simulink model "LOG_DATI_GPS_BMP_07_119_term"  (R2020b)
settings: Solver=ode4  StartTime=0.0  StopTime=Inf  FixedStep=0.02  RelTol=1e-3  EnableMultiTasking=on
PostLoadFcn:
  | , if any(exist('dsrtsu_mdlpostloadfcn', 'file') == [2, 3, 6]), try dsrtsu_mdlpostloadfcn('Execute', bdroot); catch fprintf('Error in PostLoadFcn (dsrtsu_mdlpostloadfcn) for model "%s":\n %s\n', bdroot, lasterr); end, end,
InitFcn:
  | , if any(exist('rtifpga_mdlclblib', 'file') ~= 0), rtifpga_mdlclblib('Init', bdroot); end,
values from neighbouring files (symbols this model uses):
  t_AP = 0.02    [AVVIO_AENEA_DATA.m]    (also in workspace_SFT.mat)
libraries: arduinolib x21, simulink_extras x6, svdutilitieslib x4, simulink x2
(part 3 of 3)

== matlab function LOG_DATI_GPS_BMP_07_119_term/AIR RX/MATLAB Function4 ==
  data: byte_pack input; status output; messaggio output; messaggio_2 output; byte_available input
function [status,messaggio,messaggio_2]  = Creazione_mavlink_message_2(byte_pack,byte_available)


persistent Interr_parz  message counter len_found mess_len

if isempty(Interr_parz)
    Interr_parz = false ;
end
if isempty(message)
     message = uint8(zeros(1,100 )) ;
end
if isempty (counter) 
    counter = uint8(0) ;    % variabile che conta quanti byte mancano per completare il messaggio
end 

if isempty(len_found) 
     len_found = false ;
end 

if isempty(mess_len) 
     mess_len = 0 ;
end 

status = 0;
M = length(byte_pack) ;
caso = 0 ;
messaggio = uint8(zeros(1,100 )) ;
messaggio_2 = uint8(zeros(1,100 )) ;
% LA VARIABILE INTERR_PARZ va attivata a 1 alla fine della funzone di
% lettura per indicare di leggere il successivo messaggio in arrivo 

[poss_254,num_254] = find_254(byte_pack) ;

if ((Interr_parz == true) && (num_254 == 1))                  % in questo caso verifico che il 254 sia effettivamente un altro inizio
    if (poss_254(1) ~= counter+1)
        num_254 = 0;
    end
    
end



if ( num_254 == 1 && Interr_parz == false )             
    caso = 1 ;                                                            % 1 Messaggio Intero   o parziale che inizia                % attivare alla fine della funzione Interr_parz == true o false 
elseif (num_254 == 0 && Interr_parz == true )
    caso = 2 ;                                                        % 1 Messaggio Parziale senza inizio e poi nulla 
elseif (num_254 == 1 && Interr_parz == true )                         
    caso = 3 ;                                                        % 1 Messaggio Parziale e poi un altro messaggio completo o parziale
elseif  ( num_254 == 2 && Interr_parz == false ) 
    caso = 4 ;                                                         % Due messaggi completi  oppure 1 Completo + parziale ( attivare Interr_parz alla fine del codice)
end


switch (caso)
   
    
    
    case 1
        pos_254 = poss_254(num_254) ;
        
        if pos_254 == M                                                                          % se il 254 sta alla fine
            message(1) = byte_pack(pos_254)  ;
            len_found = false ;
            Interr_parz = true ;
        else
            len = byte_pack(pos_254 + 1)  ;
            if len <= 100
                if  ((byte_pack(poss_254(1)+1) + 8) == byte_available)                                             % se abbiamo tutto il messaggio all'interno del byte_pack
                    message(1: 8 + len ) = byte_pack(pos_254 : pos_254 + (7+len) ) ;          % era cosi byte_pack(pos_254 : pos_254 + (8+len) ) ;
                    messaggio = message ;
                    status = 1 ;
                    message = uint8(zeros(1,100 )) ;
                    counter = uint8(0) ;
                    len_found = true ;
                    mess_len = 0 ;
                elseif ((byte_pack(poss_254(1)+1) + 8) > byte_available)
                    mess_len = double(byte_available) ;                                       % lunghezza del messaggio da leggere dal byte_pack ( non uguale alla lunghezza del messaggio complessivo)
                    message(1 : mess_len) = byte_pack(pos_254 : mess_len ) ;
                    len_found = true ;
                    counter = 8 + len - mess_len ;
                    Interr_parz = true ;
                end
            else
                messaggio = uint8(zeros(1,100 )) ;
                Interr_parz = false;
                message = uint8(zeros(1,100 )) ;
                counter = uint8(0) ;
                len_found = false ;
                mess_len = 0 ;
                status = 1 ;
            end
            
        end
        
        
        
        
    case 2 
        
                                     % se la lunghezza è stata trovata e quindi ho il valore di counter che indica quante componenti mancano
           if byte_pack ~= 0
                message(mess_len + 1 : mess_len + counter) = byte_pack( 1 : counter) ;
                Interr_parz = false ;
                messaggio = message ;
                status = 1 ;
                message = uint8(zeros(1,100 )) ;
                len_found = true ;
                mess_len = 0 ;
                counter = uint8(0) ;
                
           else                                                    % se ho un messaggio parziale e nello step successivo non ricevo nulla allora azzero tutto, altrimenti entro in un loop infinito di messaggi sbagliati
                Interr_parz = false ;
                messaggio = uint8(zeros(1,100)) ;
                status = 1 ;
                message = uint8(zeros(1,100 )) ;
                len_found = true ;
                mess_len = 0 ;
                counter = uint8(0) ;  
           end        
        
        

  
        
    case 3
        
        % se la lunghezza è stata trovata e quindi ho il valore di counter che indica quante componenti mancano
        pos_254 = poss_254(num_254) ;
        
        message(mess_len + 1 : mess_len + counter) = byte_pack( 1 : counter) ;
        Interr_parz = false ;
        messaggio = message ;
        status = 1 ;
        message = uint8(zeros(1,100 )) ;
        len_found = true ;
        mess_len = 0 ;
        counter = uint8(0) ;
        
        len = byte_pack(pos_254 + 1)  ;
        if len <= 100
            if  ((byte_pack(poss_254(1)+1) + 8) == uint8(byte_available-double(counter)))                                             % se abbiamo tutto il messaggio all'interno del byte_pack
                message(1: 8 + len ) = byte_pack(pos_254 : pos_254 + (7+len) ) ;          % era cosi byte_pack(pos_254 : pos_254 + (8+len) ) ;
                messaggio_2 = message ;
                status = 1 ;
                message = uint8(zeros(1,100 )) ;
                counter = uint8(0) ;
                len_found = true ;
                mess_len = 0 ;
            elseif ((byte_pack(poss_254(1)+1) + 8) > (uint8(byte_available)-counter))
                mess_len = double(byte_available) - double(counter) ;                                       % lunghezza del messaggio da leggere dal byte_pack ( non uguale alla lunghezza del messaggio complessivo)
                message(1 : mess_len) = byte_pack(pos_254 : mess_len ) ;
                len_found = true ;
                counter = 8 + len - mess_len ;
                Interr_parz = true ;
            end
        else
            messaggio = uint8(zeros(1,100 )) ;
            Interr_parz = false;
            message = uint8(zeros(1,100 )) ;
            counter = uint8(0) ;
            len_found = false ;
            mess_len = 0 ;
            status = 1 ;
        end
                
      
            
        
        
        
      
        
        
    case 4
        primo_254 = poss_254(1) ;
        secondo_254 = poss_254(2) ;
        len_primo = byte_pack(primo_254 + 1) ;
    %    messaggio(1 : len_primo + 8) = byte_pack(primo_254 : primo_254 + (len_primo + 7)) ;           %era cosi      byte_pack(primo_254 : secondo_254 - 1)  ;

        if len_primo <= 100
        messaggio(1 : len_primo + 8) = byte_pack(primo_254 : primo_254 + (len_primo + 7)) ;             %era cosi      byte_pack(primo_254 : secondo_254 - 1)  ;
        else
        messaggio = uint8(zeros(1,100 )) ;
        Interr_parz = false;
        message = uint8(zeros(1,100 )) ;
        counter = uint8(0) ;
        len_found = false ;
        mess_len = 0 ;
        end
        
        status = 1;
        
             len = byte_pack(secondo_254 + 1)  ;
             if (len <= 100 && (secondo_254-primo_254 > 3))
             if ( (byte_available - ( secondo_254))  == 7 + len    )                                         % se abbiamo tutto il messaggio all'interno del byte_pack
                message(1: 8 + len ) = byte_pack(secondo_254 : secondo_254 + (7+len) ) ;      % era cosi byte_pack(pos_254 : pos_254 + (8+len) ) ;
                messaggio_2 = message ;
                status = 2 ;
                message = uint8(zeros(1,100 )) ;
                counter = uint8(0) ;
                len_found = true ;
                mess_len = 0 ;
             else
                mess_len = length(byte_pack(secondo_254:byte_available ) ) ;    % lunghezza del messaggio da leggere dal byte_pack ( non uguale alla lunghezza del messaggio complessivo)
                message(1 : mess_len) = byte_pack(secondo_254:byte_available ) ;
                len_found = true ;
                counter = 8 + len - mess_len ;
                Interr_parz = true ;
             end
             else
               messaggio_2 = uint8(zeros(1,100 )) ;              
               Interr_parz = false;
               message = uint8(zeros(1,100 )) ;
               counter = uint8(0) ;
               len_found = false ;
               mess_len = 0 ;    
              end
             
        
        
end
end






function [position,counter] = find_254(pack) 
    position = zeros(1,3) ;
    
    M = length(pack)  ;   
    counter = 0 ;
    for i = 1 : M
        if pack(i) == 254 
            counter = counter + 1;  
            position(counter) = i; 
        end
    end
    l = pack(position(1)+1);
    if counter > 1
        if ((pack(l+8+position(1)) ~= 254) && (position(1) ~= 0))
            counter = 1;
            position(2) = 0;
        end
    end
end

== matlab function LOG_DATI_GPS_BMP_07_119_term/AIR RX/MATLAB Function2 ==
  data: mess_out output; Len output; status input; mess_1 input; mess_2 input; buff_prev input; buffer output
function [mess_out,Len,buffer] = fcn(status,mess_1,mess_2,buff_prev)


mess_out=uint8(zeros(1,100));
buffer = uint8(zeros(3,100));
counter = uint8(0);
Len = int32(0);



mess_out = buff_prev(3,:);       %il messaggio in uscita è l'ultima riga
Len = int32(mess_out(1,2));



buffer(1,:) = uint8(zeros(1,100)); %buffer è buff_prev traslato in basso di 1 riga, quindi elimino mess_out
for j=2:1:3
    buffer(j,:) = buff_prev(j-1,:);
end
i=3;
while i >= 1                        %cerco la prima riga nulla dal basso
    if buffer(i,:) == 0
        counter = uint8(i);
        break
    end
    i = i-1;
end


if status == 1
    buffer(counter,:) = mess_1;
    
elseif status == 2
    buffer(counter,:) = mess_1;
    buffer(counter-1,:) = mess_2;
    
    
else
    buffer(counter,:) = uint8(zeros(1,100));
    
    
end



end

== matlab function LOG_DATI_GPS_BMP_07_119_term/AIR RX/MATLAB Function3 ==
  data: mess_out input; new_mex output; mess_out_prev input
function new_mex = fcn(mess_out,mess_out_prev)
persistent counter

if isempty(counter)
    counter = uint16(0);
end

new_mex = uint16(0);


if ( mess_out(3) ~= mess_out_prev(3) && (all(mess_out ~= 0) == false) )

    if counter > 100
        counter = uint16(0);
    end
    counter = counter +1;
end
new_mex = counter;

end
